simulink model "comparitor"  (R2022a)
settings: Solver=VariableStepAuto  StartTime=0.0  StopTime=10.0  RelTol=1e-3
settings Model: Creator=trust  LastModifiedBy=trust

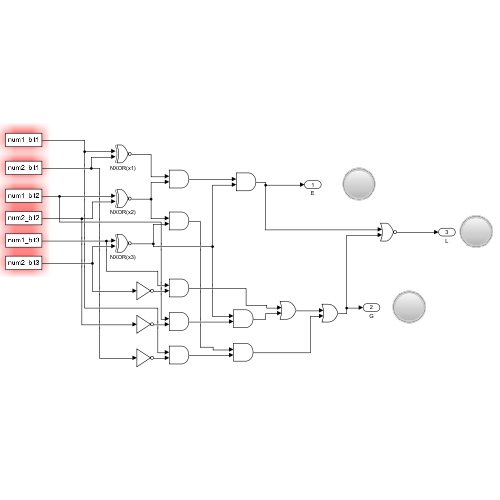
[thumbnail: Simulink's stored preview of the top-level diagram]
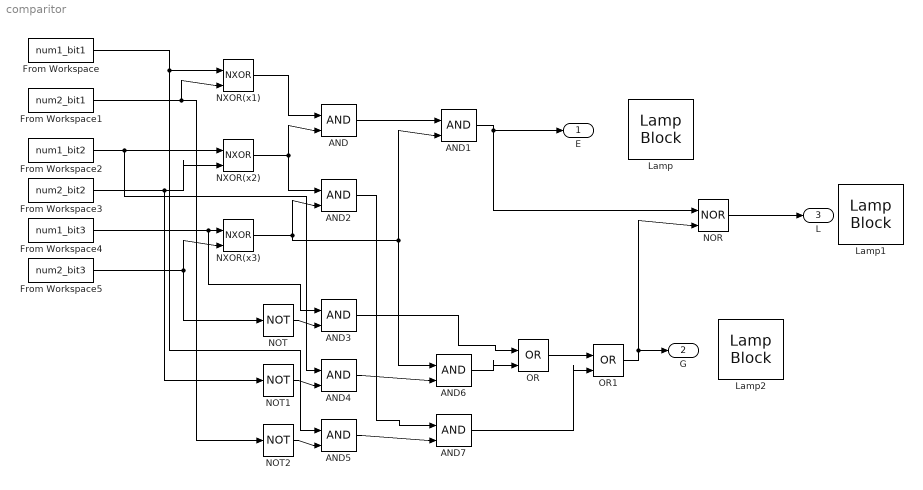
== system comparitor ==
  AND{,1..7} (8 alike) : Logic  IconShape=distinctive  AllPortsSameDT=off  OutDataTypeStr=boolean
  From Workspace : FromWorkspace  VariableName=num1_bit1
  From Workspace1 : FromWorkspace  VariableName=num2_bit1
  From Workspace2 : FromWorkspace  VariableName=num1_bit2
  From Workspace3 : FromWorkspace  VariableName=num2_bit2
  From Workspace4 : FromWorkspace  VariableName=num1_bit3
  From Workspace5 : FromWorkspace  VariableName=num2_bit3
  Lamp : LampBlock  LabelPosition=Hide
  Lamp1 : LampBlock  LabelPosition=Hide
  Lamp2 : LampBlock  LabelPosition=Hide
  NOR : Logic  Operator=NOR  IconShape=distinctive  AllPortsSameDT=off  OutDataTypeStr=boolean
  NOT : Logic  Operator=NOT  IconShape=distinctive  AllPortsSameDT=off  OutDataTypeStr=boolean
  NOT1 : Logic  Operator=NOT  IconShape=distinctive  AllPortsSameDT=off  OutDataTypeStr=boolean
  NOT2 : Logic  Operator=NOT  IconShape=distinctive  AllPortsSameDT=off  OutDataTypeStr=boolean
  NXOR(x1) : Logic  Operator=NXOR  IconShape=distinctive  AllPortsSameDT=off  OutDataTypeStr=boolean
  NXOR(x2) : Logic  Operator=NXOR  IconShape=distinctive  AllPortsSameDT=off  OutDataTypeStr=boolean
  NXOR(x3) : Logic  Operator=NXOR  IconShape=distinctive  AllPortsSameDT=off  OutDataTypeStr=boolean
  OR : Logic  Operator=OR  IconShape=distinctive  AllPortsSameDT=off  OutDataTypeStr=boolean
  OR1 : Logic  Operator=OR  IconShape=distinctive  AllPortsSameDT=off  OutDataTypeStr=boolean
  E : Outport
  G : Outport  Port=2
  L : Outport  Port=3
  wires:
  From Workspace/1 -> AND5/1, NXOR(x1)/1
  From Workspace1/1 -> NOT2/1, NXOR(x1)/2
  From Workspace2/1 -> AND4/1, NXOR(x2)/1
  From Workspace3/1 -> NOT1/1, NXOR(x2)/2
  From Workspace4/1 -> AND3/1, NXOR(x3)/1
  From Workspace5/1 -> NOT/1, NXOR(x3)/2
  NXOR(x1)/1 -> AND/1
  NXOR(x2)/1 -> AND2/1, AND/2
  NXOR(x3)/1 -> AND2/2, AND6/1, AND1/2
  AND/1 -> AND1/1
  AND1/1 -> NOR/1, E/1
  NOT/1 -> AND3/2
  NOT1/1 -> AND4/2
  NOT2/1 -> AND5/2
  AND4/1 -> AND6/2
  AND5/1 -> AND7/2
  AND2/1 -> AND7/1
  AND3/1 -> OR/1
  AND6/1 -> OR/2
  OR1/1 -> NOR/2, G/1
  NOR/1 -> L/1
  OR/1 -> OR1/1
  AND7/1 -> OR1/2
